simulink model "problem3_robotsim"  (R2021a)
settings: Solver=VariableStepAuto  StartTime=0.0  StopTime=tstop  FixedStep=1e-3
values from neighbouring files (symbols this model uses):
  f_v = [0.1 0.1 0.1 0.05 0.05 0.05]'    [problem1.m]    (also in problem3.m = zeros(6,1))
  fext = zeros(6,8)    [problem1.m]    (also in problem3.m)
  kd = [4  100   20     20   40    10]    [problem3.m]
  ki = [4  400   20     5     1      10]    [problem3.m]
  kp = [5  20     80     1     10     1]    [problem3.m]
  N = 10000    [problem3.m]
  qdes = (rand(6,1)-0.5)*2*pi    [problem3.m]
  qdotinit = zeros(6,1)    [problem1.m]    (also in problem3.m)
  qinit = zeros(6,1)    [problem1.m]    (also in problem3.m)
libraries: simulink x1, robotmaniplib x1
settings Model: Creator=wen  LastModifiedBy=Eric Tung
settings SolverCC: ZeroCrossAlgorithm=Adaptive  AlgebraicLoopSolver=TrustRegion
settings DebuggingCC: ConsistencyChecking=warning  MaxConsecutiveZCsMsg=none  MaskedZcDiagnostic=none  IgnoredZcDiagnostic=none  SFMachineParentedDataDiag=warning

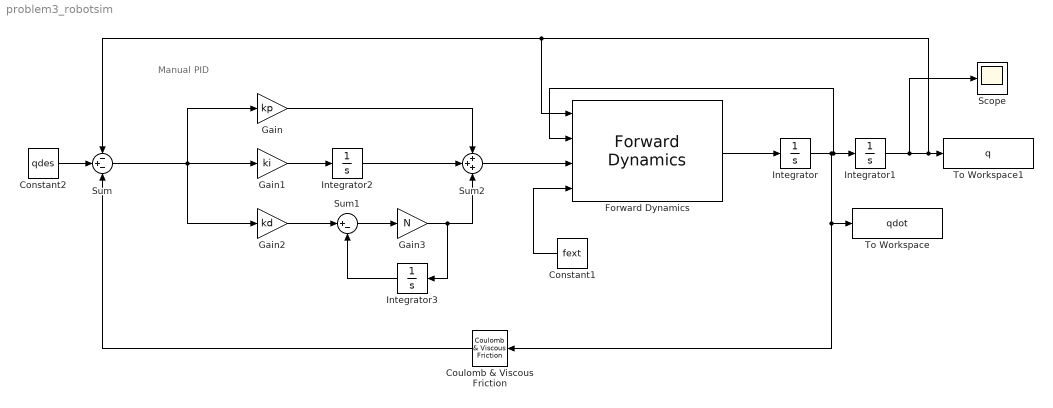
== system problem3_robotsim ==
  note: Manual PID
  Constant1 : Constant  Value=fext
  Constant2 : Constant  Value=qdes
  Coulomb & Viscous Friction : simulink/Discontinuities/Coulomb & Viscous Friction  offset=f_c  gain=f_v
  Forward Dynamics : robotmaniplib/Forward Dynamics  RigidBodyTree=abb  SimulateUsing=Interpreted execution
  Gain : Gain  Gain=kp
  Gain1 : Gain  Gain=ki
  Gain2 : Gain  Gain=kd
  Gain3 : Gain  Gain=N
  Integrator : Integrator  InitialCondition=qdotinit
  Integrator1 : Integrator  InitialCondition=qinit
  Integrator2 : Integrator
  Integrator3 : Integrator
  Scope : Scope
  Sum : Sum  Inputs=-+-
  Sum1 : Sum  Inputs=|+-
  Sum2 : Sum  Inputs=+++
  To Workspace : ToWorkspace  VariableName=qdot  SampleTime=-1
  To Workspace1 : ToWorkspace  VariableName=q  SampleTime=-1
  wires:
  Forward Dynamics/1 -> Integrator/1
  Integrator/1 -> Coulomb & Viscous Friction/1, To Workspace/1, Forward Dynamics/2, Integrator1/1
  Integrator1/1 -> Sum/1, Forward Dynamics/1, To Workspace1/1, Scope/1
  Constant1/1 -> Forward Dynamics/4
  Constant2/1 -> Sum/2
  Sum2/1 -> Forward Dynamics/3
  Coulomb & Viscous Friction/1 -> Sum/3
  Gain1/1 -> Integrator2/1
  Gain3/1 -> Integrator3/1, Sum2/3
  Integrator2/1 -> Sum2/2
  Gain2/1 -> Sum1/1
  Integrator3/1 -> Sum1/2
  Gain/1 -> Sum2/1
  Sum1/1 -> Gain3/1
  Sum/1 -> Gain2/1, Gain/1, Gain1/1
